simulink model "Darko_long"  (R2026a)
settings: Solver=VariableStepAuto
values from neighbouring files (symbols this model uses):
  delta_inertia = 0    [DARKO_MAIN.m]    (also in DARKO_MAIN_long.m; check_Darko_long.m)
  delta_mass = 0    [DARKO_MAIN.m]    (also in DARKO_MAIN_long.m; check_Darko_long.m)
  delta_phi_coef = 0.0    (= 0)    [DARKO_MAIN.m]    (also in DARKO_MAIN_long.m; check_Darko_long.m)
  time_var_param = 13500    [DARKO_MAIN.m]    (also in DARKO_MAIN_long.m = inf; check_Darko_long.m = inf)
  Ts = 1/500    (= 0.002)    [DARKO_MAIN.m]    (also in DARKO_MAIN_long.m; check_Darko_long.m)
  xj0 = [vb; wb; q]    [DARKO_MAIN.m]    (also in DARKO_MAIN_long.m = xts(:, trim_sol); check_Darko_long.m = xt)
libraries: sharedtransform x1
settings Model: Creator=devinbellll  LastModifiedBy=devinbellll

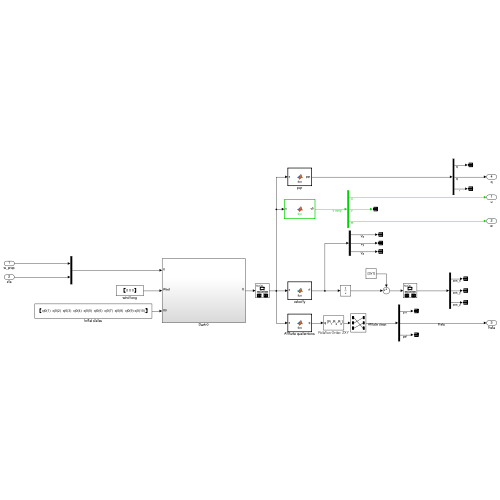
[thumbnail: Simulink's stored preview of the top-level diagram]
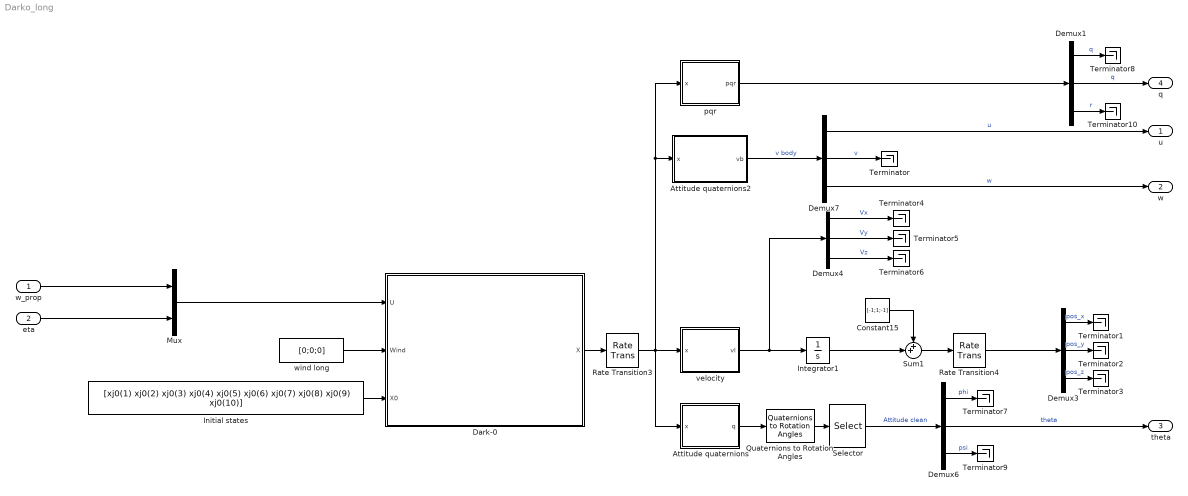
== system Darko_long ==
  w_prop : Inport
  eta : Inport  Port=2
  Attitude quaternions : MATLAB Function  TreatAsAtomicUnit=on
  Attitude quaternions2 : MATLAB Function  TreatAsAtomicUnit=on
  Constant15 : Constant  Value=[-1;1;-1]  SampleTime=Ts
  Dark-0 : Subsystem
  Demux{1,3..4,6..7} (5 alike) : Demux  Outputs=3
  Initial states : Constant  Value=[xj0(1) xj0(2) xj0(3) xj0(4) xj0(5) xj0(6) xj0(7) xj0(8) xj0(9) xj0(10)]  SampleTime=Ts
  Integrator1 : Integrator  InitialCondition=[1;-1;1.20]
  Mux : Mux  Inputs=2
  Quaternions to Rotation Angles : sharedtransform/Quaternions to Rotation Angles  rotationOrder=ZXY  aMode=aMode
  Rate Transition3 : RateTransition  OutPortSampleTime=Ts
  Rate Transition4 : RateTransition  OutPortSampleTime=Ts
  Selector : Selector  InputPortWidth=3  IndexOptions=Index vector (dialog)  Indices=[2 3 1]  OutputSizes=1
  Sum1 : Sum  Inputs=++|
  Terminator{,1..10} (11 alike) : Terminator
  pqr : MATLAB Function  TreatAsAtomicUnit=on
  velocity : MATLAB Function  TreatAsAtomicUnit=on
  wind long : Constant  Value=[0;0;0]
  u : Outport
  w : Outport  Port=2
  theta : Outport  Port=3
  q : Outport  Port=4
  wires:
  pqr/1(pqr) -> Demux1/1
  Demux4/1 -> Terminator4/1  "Vx"
  Demux6/2 -> theta/1  "theta"
  Constant15/1 -> Sum1/1
  Integrator1/1 -> Sum1/2
  Demux7/1 -> u/1  "u"
  Demux4/2 -> Terminator5/1  "Vy"
  Demux6/3 -> Terminator9/1  "psi"
  Rate Transition4/1 -> Demux3/1
  Demux6/1 -> Terminator7/1  "phi"
  Sum1/1 -> Rate Transition4/1
  velocity/1(vl) -> Integrator1/1, Demux4/1
  Quaternions to Rotation Angles/1 -> Selector/1
  Attitude quaternions/1(q) -> Quaternions to Rotation Angles/1
  Demux4/3 -> Terminator6/1  "Vz"
  Attitude quaternions2/1(vb) -> Demux7/1  "v body"
  Initial states/1 -> Dark-0/3(X0)
  Rate Transition3/1 -> Attitude quaternions/1(x), velocity/1(x), pqr/1(x), Attitude quaternions2/1(x)
  Dark-0/1(X) -> Rate Transition3/1
  Selector/1 -> Demux6/1  "Attitude clean"
  Mux/1 -> Dark-0/1(U)
  wind long/1 -> Dark-0/2(Wind)
  Demux7/3 -> w/1  "w"
  Demux7/2 -> Terminator/1  "v"
  Demux3/1 -> Terminator1/1  "pos_x"
  Demux3/2 -> Terminator2/1  "pos_y"
  Demux3/3 -> Terminator3/1  "pos_z"
  Demux1/2 -> q/1  "q"
  Demux1/1 -> Terminator8/1  "q"
  Demux1/3 -> Terminator10/1  "r"
  w_prop/1 -> Mux/1
  eta/1 -> Mux/2

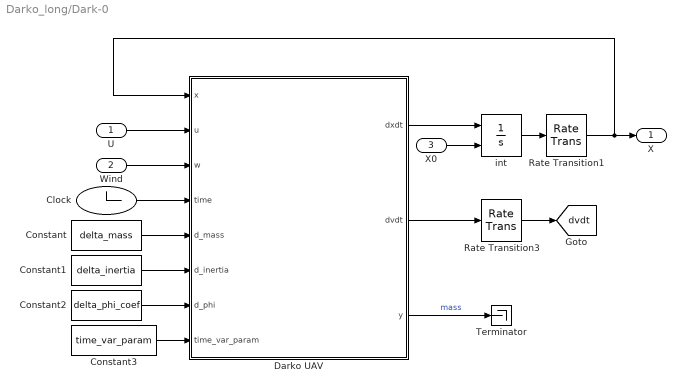
== system Darko_long/Dark-0 ==
  U : Inport
  Wind : Inport  Port=2
  X0 : Inport  Port=3
  Clock : Clock
  Constant : Constant  Value=delta_mass  SampleTime=Ts
  Constant1 : Constant  Value=delta_inertia  SampleTime=Ts
  Constant2 : Constant  Value=delta_phi_coef  SampleTime=Ts
  Constant3 : Constant  Value=time_var_param  SampleTime=Ts
  Darko UAV : MATLAB Function  TreatAsAtomicUnit=on
  Rate Transition1 : RateTransition  OutPortSampleTime=Ts
  Rate Transition3 : RateTransition  OutPortSampleTime=Ts
  Terminator : Terminator
  int : Integrator  InitialConditionSource=external
  X : Outport  VectorParamsAs1DForOutWhenUnconnected=off
  tag scope: dvdt=global
  wires:
  U/1 -> Darko UAV/2(u)
  Darko UAV/1(dxdt) -> int/1
  Wind/1 -> Darko UAV/3(w)
  X0/1 -> int/2
  Darko UAV/2(dvdt) -> Rate Transition3/1
  Rate Transition3/1 -> [dvdt]
  int/1 -> Rate Transition1/1
  Rate Transition1/1 -> X/1, Darko UAV/1(x)
  Clock/1 -> Darko UAV/4(time)
  Constant/1 -> Darko UAV/5(d_mass)
  Constant2/1 -> Darko UAV/7(d_phi)
  Constant1/1 -> Darko UAV/6(d_inertia)
  Darko UAV/3(y) -> Terminator/1  "mass"
  Constant3/1 -> Darko UAV/8(time_var_param)

== matlab function Darko_long/Attitude quaternions ==
  data: x input; q output
function q  = fcn(x)
%#codegen

%% quaternion computation
q = x(7:10);

== matlab function Darko_long/Dark-0/Darko UAV ==
  data: x input; u input; dxdt output; w input; dvdt output; time input; d_mass input; d_inertia input; d_phi input; time_var_param input; y output
function [dxdt, dvdt,y] = fcn(x, u, w, time, d_mass, d_inertia, d_phi, time_var_param)
%#codegen

drone = generateDarko();

% parameter perturbation for robustness tests: switched on when
% time > time_var_param (s); amounts set by delta_* workspace variables
if(time > time_var_param)
    drone.MASS    = drone.MASS + d_mass*drone.MASS;
    drone.INERTIA = drone.INERTIA + d_inertia*drone.INERTIA;
    drone.PHI     = drone.PHI + d_phi*drone.PHI;
end
y = drone.MASS;

dxdt = sysEqt_long(x, u, w, drone);
dvdt = dxdt(1:3);

== matlab function Darko_long/velocity ==
  data: x input; vl output
function vl  = fcn(x)
%#codegen

vl = x(1:3);
%q  = x(7:10,1);
%D = q2dcm(q');

%vb = D*vl;
%vb(3) = -vb(3); % NED coordinate

%vl(3) = -x(3);

== matlab function Darko_long/Attitude quaternions2 ==
  data: x input; vb output
function vb   = fcn(x)
%#codegen

vl = x(1:3);
%% quaternion and DCM computation
q  = x(7:10,1);
D = q2dcm(q');


%% speed in body-frame
vb = D*vl;

== matlab function Darko_long/pqr ==
  data: x input; pqr output
function pqr  = fcn(x)
%#codegen

pqr = x(4:6);
